simulink model "SD2231_Lab1_2022"  (R2020b)
settings: Solver=VariableStepAuto  StartTime=0.0  StopTime=inf  RelTol=1e-3
values from neighbouring files (symbols this model uses):
  delay = 250    [initial.m]
  K_awup = Ki_br_r/Kp_br_r    (= 10.4166666667)    [initial.m]
  K_brake = K_brake(3)    [initial.m]
  K_em = K_em(3)    [initial.m]
  Kd_br_f = 0*0.6*T_new_rl_b    (= 0)    [initial.m]
  Kd_br_r = 0.6*T_new_rl_b    (= 0.1722)    [initial.m]
  Kd_tr = 0.6*T_new    (= 0.0093)    [initial.m]
  Ki_br_f = 0.5*0.6*T_new_rl_b/L_new_rl_b^2    (= 37.3697916667)    [initial.m]
  Ki_br_r = 0.6*T_new_rl_b/L_new_rl_b^2    (= 74.7395833333)    [initial.m]
  Ki_tr = 0.6*T_new/L_new^2    (= 4.12188365651)    [initial.m]
  Kp_br_f = 1.2*T_new_rl_b/L_new_rl_b    (= 7.175)    [initial.m]
  Kp_br_r = 1.2*T_new_rl_b/L_new_rl_b    (= 7.175)    [initial.m]
  Kp_tr = 2.2*1.2*T_new/L_new    (= 0.861473684211)    [initial.m]
  N = 100    [initial.m]
  ref_br_f = 0.15    [initial.m]
  ref_br_r = 0.17-0.1    (= 0.07)    [initial.m]
  ref_tr = 0.06    [initial.m]
  step_time = 2    [initial.m]
  threshold_br_f = ref_br_f-0.05    (= 0.1)    [initial.m]
  threshold_br_r = ref_br_r-0.05    (= 0.02)    [initial.m]
  threshold_tc = ref_tr-0.02    (= 0.04)    [initial.m]
  vx_threshold = 1    [initial.m]
undefined symbols (not defined in the file or in its folder): DiscIntNeverNeededParam, Veh
libraries: CarMaker4SL x38, simulink x2, autolibmappedmotor x2
(part 2 of 4)

== system SD2231_Lab1_2022/CarMaker/Your ABS Controller/Activation Logic Br RR ==
  Brake Pedal : Inport
  vx : Inport  Port=2
  <Vehicle ax> : Inport  Port=3
  " Slip" : Inport  Port=4
  AdjBr FL : Scope  NumInputPorts=2
  Constant : Constant  Value=threshold_br_r
  Constant1 : Constant  Value=vx_threshold
  MATLAB Function : MATLAB Function  TreatAsAtomicUnit=on
  Subsystem : Subsystem
      settings: PortSchema="{\"entries\":[{\"content\":{\"sides\":[{\"content\":{\"connectorIds\":[\"In1\",\"In2\"]},\"type\":\"ConnectorPlacement.EquallySpacedRectSide\",\"uuid\":\"5cbd211e-f9c8-43f4-83d7-871b04fe90ea\"},{\"content\":{\"connectorIds\":[\"Out1\"],\"side\":\"RIGHT\"},\"type\":\"ConnectorPlacement.EquallySpacedRectSide\",\"uuid\":\"7fa8af9f-7b9f-4089-80e3-a9aa0072d831\"},{\"content\":{\"connectorIds\":[\"In3\"],\"side\":\"TOP\"},\"type\":\"ConnectorPlacement.EquallySpacedRectSide\",\"uuid\":\"e4a0fb24-cce3-4d5d-8c82-dcee69222b7b\"},{\"content\":{\"connectorIds\":[],\"side\":\"HIDDEN\"},\"type\":\"ConnectorPlacement.EquallySpacedRectSide\",\"uuid\":\"1dbaf2b9-056b-4908-bf5e-3fea819f12fb\"}]},\"type\":\"ConnectorPlacement.EquallySpacedConnector\",\"uuid\":\"c1423465-905b-4b91-a244-d319c117cff2\"}],\"packageUris\":[\"http://schema.mathworks.com/mf0/Connector/R2020b\"],\"version\":\"1.0\"}"
  ref : Constant  Value=ref_br_r
  BrkAdjust : Outport
  wires:
  Constant1/1 -> MATLAB Function/7(vx_threshold)
  ref/1 -> Subsystem/2(ref_slip)
  MATLAB Function/1(y) -> BrkAdjust/1, AdjBr FL/1
  Subsystem/1(AdjBr) -> MATLAB Function/5(AdjBrk)
  " Slip"/1 -> MATLAB Function/4(slip), Subsystem/1(slip)
  Brake Pedal/1 -> MATLAB Function/3(Brk), Subsystem/3(Brake Pedal), AdjBr FL/2
  Constant/1 -> MATLAB Function/6(threshold)
  <Vehicle ax>/1 -> MATLAB Function/2(ax)
  vx/1 -> MATLAB Function/1(vx)

== system SD2231_Lab1_2022/CarMaker/Your ABS Controller/Activation Logic Br RR old 2 ==
  Brake Pedal : Inport
  vx : Inport  Port=2
  <Vehicle ax> : Inport  Port=3
  " Slip" : Inport  Port=4
  AdjBr RR : Scope  NumInputPorts=2
  Constant : Constant  Value=threshold_br_r
  Constant1 : Constant  Value=vx_threshold
  Controller : Subsystem
      settings: PortSchema="{\"entries\":[{\"content\":{\"sides\":[{\"content\":{\"connectorIds\":[\"In1\",\"In2\"]},\"type\":\"ConnectorPlacement.EquallySpacedRectSide\",\"uuid\":\"5cec5cc2-4d6d-4b1d-b966-22042b341a0b\"},{\"content\":{\"connectorIds\":[\"Out1\"],\"side\":\"RIGHT\"},\"type\":\"ConnectorPlacement.EquallySpacedRectSide\",\"uuid\":\"00dd4905-e656-4dce-9ac4-4fe3f823c1f7\"},{\"content\":{\"connectorIds\":[\"In3\"],\"side\":\"TOP\"},\"type\":\"ConnectorPlacement.EquallySpacedRectSide\",\"uuid\":\"696fd126-3e4c-4262-b5bc-c3625537c515\"},{\"content\":{\"connectorIds\":[],\"side\":\"HIDDEN\"},\"type\":\"ConnectorPlacement.EquallySpacedRectSide\",\"uuid\":\"3dd45ed5-25e2-4347-abdf-21481b15662e\"}]},\"type\":\"ConnectorPlacement.EquallySpacedConnector\",\"uuid\":\"5000242c-67c6-4855-a207-79a064e97cc6\"}],\"packageUris\":[\"http://schema.mathworks.com/mf0/Connector/R2020b\"],\"version\":\"1.0\"}"
  MATLAB Function : MATLAB Function  TreatAsAtomicUnit=on
  Switch : Switch  Commented=on  Criteria=u2 > Threshold  Threshold=5
  ref : Constant  Value=ref_br_r
  ref1 : Constant  Commented=on  Value=0
  BrkAdjust : Outport
  tag scope: ref_br=global
  wires:
  <Vehicle ax>/1 -> MATLAB Function/2(ax)
  Constant/1 -> MATLAB Function/6(threshold)
  Brake Pedal/1 -> AdjBr RR/2, Controller/3(Brake Pedal), MATLAB Function/3(Brk)
  " Slip"/1 -> Controller/1(slip), MATLAB Function/4(slip)
  Controller/1(AdjThr) -> MATLAB Function/5(AdjBrk)
  MATLAB Function/1(y) -> BrkAdjust/1, AdjBr RR/1
  ref/1 -> Controller/2(ref_slip), [ref_br]
  vx/1 -> MATLAB Function/1(vx)
  Constant1/1 -> MATLAB Function/7(vx_threshold)
  ? -> Switch/2
  Switch/1 -> ?
  ref1/1 -> Switch/3

== system SD2231_Lab1_2022/CarMaker/Your ABS Controller/Activation Logic1 ==
  Brake Pedal : Inport
  vx : Inport  Port=2
  <Vehicle ax> : Inport  Port=3
  " Slip" : Inport  Port=4
  Constant : Constant  Value=threshold_br_f
  MATLAB Function : MATLAB Function  Commented=on  TreatAsAtomicUnit=on
  MATLAB Function1 : MATLAB Function  TreatAsAtomicUnit=on
  Scope : Scope
  Scope1 : Scope
  Subsystem : Subsystem  Commented=on
  Subsystem1 : Subsystem
      settings: PortSchema="{\"entries\":[{\"content\":{\"sides\":[{\"content\":{\"connectorIds\":[\"In1\",\"In2\"]},\"type\":\"ConnectorPlacement.EquallySpacedRectSide\",\"uuid\":\"8c5c4b92-db61-456f-8d74-c8cf023ef126\"},{\"content\":{\"connectorIds\":[\"Out1\"],\"side\":\"RIGHT\"},\"type\":\"ConnectorPlacement.EquallySpacedRectSide\",\"uuid\":\"6d2f9992-79bb-457d-890b-805505bdee0e\"},{\"content\":{\"connectorIds\":[],\"side\":\"TOP\"},\"type\":\"ConnectorPlacement.EquallySpacedRectSide\",\"uuid\":\"0d630a28-683f-44cf-bfe5-2a203886c9bc\"},{\"content\":{\"connectorIds\":[\"In3\"],\"side\":\"BOTTOM\"},\"type\":\"ConnectorPlacement.EquallySpacedRectSide\",\"uuid\":\"65c4d467-3a6d-4ab0-8a2a-27ecddcdb5a7\"},{\"content\":{\"connectorIds\":[],\"side\":\"HIDDEN\"},\"type\":\"ConnectorPlacement.EquallySpacedRectSide\",\"uuid\":\"17dfa9f0-a896-4b0a-816c-6439308f7c21\"}]},\"type\":\"ConnectorPlacement.EquallySpacedConnector\",\"uuid\":\"38ebf0b2-c1be-4567-9f2f-ae9c854cb505\"}],\"packageUris\":[\"http://schema.mathworks.com/mf0/Connector/R2020b\"],\"version\":\"1.0\"}"
  Switch : Switch  Criteria=u2 > Threshold  Threshold=0.5
  ref : Constant  Value=ref_br_f
  BrkAdjust : Outport
  wires:
  Constant/1 -> MATLAB Function1/4(threshold)
  ref/1 -> Subsystem1/2(ref_slip)
  MATLAB Function1/1(s) -> Subsystem1/1(slip)
  " Slip"/1 -> MATLAB Function1/3(slip)
  MATLAB Function1/2(y) -> Scope/1, Subsystem1/3(y), Switch/2
  Brake Pedal/1 -> Switch/3, MATLAB Function1/5(Brk)
  Subsystem/1(AdjThr) -> MATLAB Function/5(AdjBrk)
  <Vehicle ax>/1 -> MATLAB Function1/1(ax)
  vx/1 -> MATLAB Function1/2(vx)
  ? -> Subsystem/1(slip), MATLAB Function/4(slip)
  Subsystem1/1(AdjThr) -> Switch/1
  Switch/1 -> Scope1/1, BrkAdjust/1

== system SD2231_Lab1_2022/CarMaker/Your Traction Controller/Activation Logic RL tr1 ==
  Thr : Inport
  vx : Inport  Port=2
  <Vehicle ax> : Inport  Port=3
  " Slip" : Inport  Port=4
  Constant : Constant  Value=threshold_tc
  If : If  IfExpression=u1 > 0.5
  If Action Subsystem : Subsystem  TreatAsAtomicUnit=on
  MATLAB Function : MATLAB Function  Commented=on  TreatAsAtomicUnit=on
  MATLAB Function1 : MATLAB Function  TreatAsAtomicUnit=on
  Merge : Merge
  Scope : Scope
  Scope1 : Scope
  Subsystem : Subsystem  Commented=on
  Subsystem1 : Subsystem
  ref : Constant  Value=ref_tr
  y tracking RL tr : Scope
  AdjThr : Outport
  wires:
  Merge/1 -> AdjThr/1, Scope/1
  If Action Subsystem/1(Out1) -> Merge/2
  If/2 -> If Action Subsystem/Action
  If/1 -> Subsystem1/Action
  Subsystem1/1(AdjThr) -> Merge/1
  ? -> MATLAB Function/4(slip), Subsystem/1(slip)
  vx/1 -> MATLAB Function1/2(vx)
  <Vehicle ax>/1 -> MATLAB Function1/1(ax)
  Subsystem/1(AdjThr) -> MATLAB Function/5(AdjBrk)
  Thr/1 -> MATLAB Function1/5(Thr), Subsystem1/3(Thr), If Action Subsystem/1(Throttle), Scope1/1
  MATLAB Function1/2(y) -> If/1, y tracking RL tr/1
  " Slip"/1 -> MATLAB Function1/3(slip)
  MATLAB Function1/1(s) -> Subsystem1/1(slip)
  ref/1 -> Subsystem1/2(ref_slip)
  Constant/1 -> MATLAB Function1/4(threshold)

== system SD2231_Lab1_2022/CarMaker/Your Traction Controller/Activation Logic RL tr2 ==
  Thr : Inport
  vx : Inport  Port=2
  <Vehicle ax> : Inport  Port=3
  " Slip" : Inport  Port=4
  Add : Sum
  Constant : Constant  Value=threshold_tc
  MATLAB Function : MATLAB Function  Commented=on  TreatAsAtomicUnit=on
  MATLAB Function1 : MATLAB Function  TreatAsAtomicUnit=on
  Subsystem : Subsystem  Commented=on
  Subsystem2 : Subsystem
  ref1 : Constant  Value=ref_tr
  AdjThr : Outport
  wires:
  ? -> MATLAB Function/4(slip), Subsystem/1(slip)
  vx/1 -> MATLAB Function1/2(vx)
  <Vehicle ax>/1 -> MATLAB Function1/1(ax)
  Subsystem/1(AdjThr) -> MATLAB Function/5(AdjBrk)
  Thr/1 -> Add/2, MATLAB Function1/5(Thr)
  " Slip"/1 -> MATLAB Function1/3(slip)
  Constant/1 -> MATLAB Function1/4(threshold)
  ref1/1 -> Subsystem2/2(ref_slip)
  Subsystem2/1(AdjThr) -> Add/1
  Add/1 -> AdjThr/1
  ? -> Subsystem2/1(slip)

== system SD2231_Lab1_2022/CarMaker/Your Traction Controller/Activation Logic Tr RL ==
  <Throttle> : Inport
  ax : Inport  Port=2
  <RL Slip> : Inport  Port=3
  AdjTh RL : Scope
  Constant : Constant  Value=threshold_tc
  Delay : Delay  Commented=on  DelayLength=delay
  MATLAB Function : MATLAB Function  TreatAsAtomicUnit=on
  Subsystem : Subsystem
      settings: PortSchema="{\"entries\":[{\"content\":{\"sides\":[{\"content\":{\"connectorIds\":[\"In1\",\"In2\"]},\"type\":\"ConnectorPlacement.EquallySpacedRectSide\",\"uuid\":\"79f5dd27-5b3e-419d-80a6-0989bf4121ab\"},{\"content\":{\"connectorIds\":[\"Out1\"],\"side\":\"RIGHT\"},\"type\":\"ConnectorPlacement.EquallySpacedRectSide\",\"uuid\":\"49c92f03-337c-4fd9-9025-501eb5f091b3\"},{\"content\":{\"connectorIds\":[\"In3\"],\"side\":\"TOP\"},\"type\":\"ConnectorPlacement.EquallySpacedRectSide\",\"uuid\":\"f0086f1c-5e21-497a-b605-cecce1a91be6\"},{\"content\":{\"connectorIds\":[],\"side\":\"HIDDEN\"},\"type\":\"ConnectorPlacement.EquallySpacedRectSide\",\"uuid\":\"c7823733-75a9-46f7-a877-dbd7359ce4af\"}]},\"type\":\"ConnectorPlacement.EquallySpacedConnector\",\"uuid\":\"cd50cf1a-1747-4545-b326-76b9fad2c095\"}],\"packageUris\":[\"http://schema.mathworks.com/mf0/Connector/R2020b\"],\"version\":\"1.0\"}"
  ref : Constant  Value=ref_tr
  y tracking RR : Scope
  RLTrqAdjust : Outport
  wires:
  Subsystem/1(AdjThr) -> MATLAB Function/4(AdjThr)
  MATLAB Function/2(dbg) -> y tracking RR/1
  ax/1 -> MATLAB Function/1(ax)
  Constant/1 -> MATLAB Function/5(threshold)
  <Throttle>/1 -> Subsystem/3(<Throttle>), MATLAB Function/2(Thr)
  <RL Slip>/1 -> Subsystem/1(slip), MATLAB Function/3(slip)
  MATLAB Function/1(y) -> AdjTh RL/1, RLTrqAdjust/1
  ref/1 -> Subsystem/2(ref_slip)

== system SD2231_Lab1_2022/CarMaker/Your Traction Controller/Activation Logic Tr RR ==
  Thr : Inport
  <Vehicle ax> : Inport  Port=2
  " Slip" : Inport  Port=3
  AdjTh RR : Scope
  Constant : Constant  Value=threshold_tc
  Controller : Subsystem  Commented=on
      settings: PortSchema="{\"entries\":[{\"content\":{\"sides\":[{\"content\":{\"connectorIds\":[\"In1\",\"In2\"]},\"type\":\"ConnectorPlacement.EquallySpacedRectSide\",\"uuid\":\"52813697-ab49-4c87-b189-f3c4bbd3a435\"},{\"content\":{\"connectorIds\":[\"Out1\"],\"side\":\"RIGHT\"},\"type\":\"ConnectorPlacement.EquallySpacedRectSide\",\"uuid\":\"31f7970c-8430-4628-a4a3-49e1cbd89ba0\"},{\"content\":{\"connectorIds\":[\"In3\"],\"side\":\"TOP\"},\"type\":\"ConnectorPlacement.EquallySpacedRectSide\",\"uuid\":\"62e35f04-27eb-4615-837d-613f48d08a05\"},{\"content\":{\"connectorIds\":[],\"side\":\"HIDDEN\"},\"type\":\"ConnectorPlacement.EquallySpacedRectSide\",\"uuid\":\"731c0a9f-c9f4-41b7-8d96-4f2cebcab437\"}]},\"type\":\"ConnectorPlacement.EquallySpacedConnector\",\"uuid\":\"9bef8a7f-94a8-4a01-95b1-5b9f04346e26\"}],\"packageUris\":[\"http://schema.mathworks.com/mf0/Connector/R2020b\"],\"version\":\"1.0\"}"
  MATLAB Function : MATLAB Function  TreatAsAtomicUnit=on
  Subsystem : Subsystem
      settings: PortSchema="{\"entries\":[{\"content\":{\"sides\":[{\"content\":{\"connectorIds\":[\"In1\",\"In2\"]},\"type\":\"ConnectorPlacement.EquallySpacedRectSide\",\"uuid\":\"79f5dd27-5b3e-419d-80a6-0989bf4121ab\"},{\"content\":{\"connectorIds\":[\"Out1\"],\"side\":\"RIGHT\"},\"type\":\"ConnectorPlacement.EquallySpacedRectSide\",\"uuid\":\"49c92f03-337c-4fd9-9025-501eb5f091b3\"},{\"content\":{\"connectorIds\":[\"In3\"],\"side\":\"TOP\"},\"type\":\"ConnectorPlacement.EquallySpacedRectSide\",\"uuid\":\"f0086f1c-5e21-497a-b605-cecce1a91be6\"},{\"content\":{\"connectorIds\":[],\"side\":\"HIDDEN\"},\"type\":\"ConnectorPlacement.EquallySpacedRectSide\",\"uuid\":\"c7823733-75a9-46f7-a877-dbd7359ce4af\"}]},\"type\":\"ConnectorPlacement.EquallySpacedConnector\",\"uuid\":\"cd50cf1a-1747-4545-b326-76b9fad2c095\"}],\"packageUris\":[\"http://schema.mathworks.com/mf0/Connector/R2020b\"],\"version\":\"1.0\"}"
  ref : Constant  Value=ref_tr
  ThrAdjust : Outport
  wires:
  <Vehicle ax>/1 -> MATLAB Function/1(ax)
  Constant/1 -> MATLAB Function/5(threshold)
  Thr/1 -> Subsystem/3(<Throttle>), MATLAB Function/2(Thr)
  " Slip"/1 -> Subsystem/1(slip), MATLAB Function/3(slip)
  Subsystem/1(AdjThr) -> MATLAB Function/4(AdjThr)
  MATLAB Function/1(y) -> AdjTh RR/1, ThrAdjust/1
  ref/1 -> Subsystem/2(ref_slip)

== system SD2231_Lab1_2022/CarMaker/Your Traction Controller/Activation Logic1 ==
  <Throttle> : Inport
  <Vehicle ax> : Inport  Port=2
  <RL Slip> : Inport  Port=3
  Constant : Constant  Value=threshold_tc
  MATLAB Function : MATLAB Function  TreatAsAtomicUnit=on
  Subsystem : Subsystem
  ref : Constant  Value=ref_tr
  TrqAdjust : Outport
  wires:
  <Throttle>/1 -> MATLAB Function/2(Thr)
  <RL Slip>/1 -> Subsystem/1(slip), MATLAB Function/3(slip)
  Subsystem/1(AdjThr) -> MATLAB Function/4(AdjThr)
  ref/1 -> Subsystem/2(ref_slip)
  Constant/1 -> MATLAB Function/5(threshold)
  MATLAB Function/1(y) -> TrqAdjust/1
  <Vehicle ax>/1 -> MATLAB Function/1(ax)

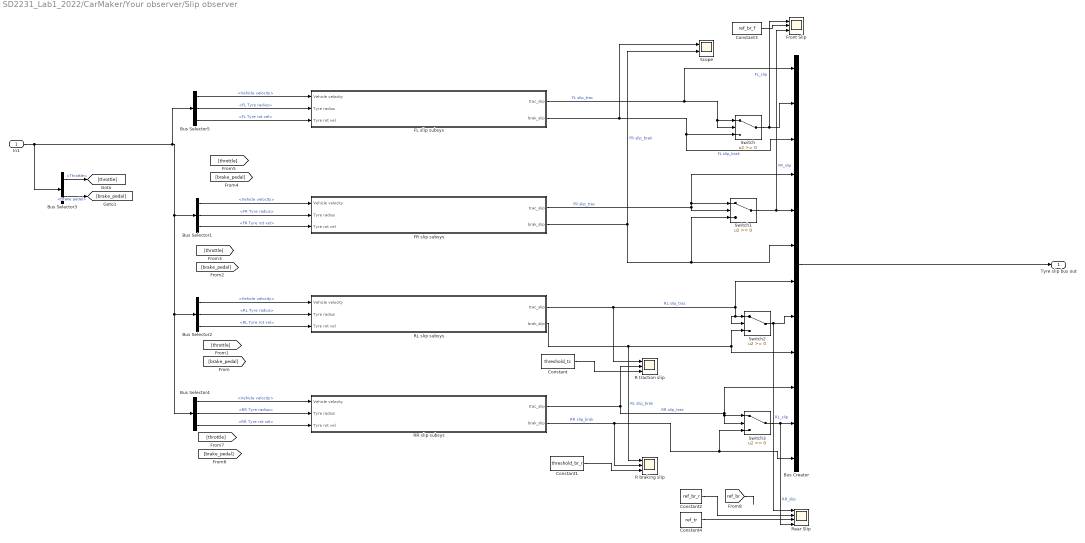
== system SD2231_Lab1_2022/CarMaker/Your observer/Slip observer ==
  In1 : Inport
  " FL slip subsys" : Subsystem
  " FR slip subsys" : Subsystem
  " RL slip subsys" : Subsystem
  " RR slip subsys" : Subsystem
  Bus Creator : BusCreator  Inputs=12
  Bus Selector1 : BusSelector  OutputSignals=Vehicle velocity,FR Tyre radius,FR Tyre rot vel
  Bus Selector2 : BusSelector  OutputSignals=Vehicle velocity,RL Tyre radius,RL Tyre rot vel
  Bus Selector3 : BusSelector  OutputSignals=Throttle,Brake pedal
  Bus Selector4 : BusSelector  OutputSignals=Vehicle velocity,RR Tyre radius,RR Tyre rot vel
  Bus Selector5 : BusSelector  OutputSignals=Vehicle velocity,FL Tyre radius,FL Tyre rot vel
  Constant : Constant  Value=threshold_tc
  Constant1 : Constant  Value=threshold_br_r
  Constant2 : Constant  Value=ref_br_r
  Constant3 : Constant  Value=ref_br_f
  Constant4 : Constant  Value=ref_tr
  Front Slip : Scope  NumInputPorts=3
  R braking slip : Scope  NumInputPorts=3
  R traction slip : Scope  NumInputPorts=3
  Rear Slip : Scope  NumInputPorts=4
  Scope : Scope  NumInputPorts=2
  Switch{,1..3} (4 alike) : Switch
  Tyre slip bus out : Outport
  wires:
  Bus Selector3/1 -> [throttle]  "<Throttle>"
  Bus Selector3/2 -> [brake_pedal]  "<Brake pedal>"
  Bus Selector4/1 -> " RR slip subsys"/1(Vehicle velocity)  "<Vehicle velocity>"
  Bus Selector4/2 -> " RR slip subsys"/2(" Tyre radius")  "<RR Tyre radius>"
  Bus Selector4/3 -> " RR slip subsys"/3(Tyre rot vel)  "<RR Tyre rot vel>"
  " FL slip subsys"/1(trac_slip) -> Switch/2, Switch/1, Bus Creator/1  "FL slip_trac"
  " FL slip subsys"/2(brak_slip) -> Scope/1, Bus Creator/3, Switch/3  "FL slip_brak"
  " RL slip subsys"/2(brak_slip) -> R braking slip/1, Bus Creator/9, Switch2/3  "RL slip_brak"
  " RL slip subsys"/1(trac_slip) -> Switch2/2, Switch2/1, Bus Creator/7, R traction slip/1  "RL slip_trac"
  " RR slip subsys"/1(trac_slip) -> R traction slip/2, Switch3/2, Switch3/1, Bus Creator/10  "RR slip_trac"
  " RR slip subsys"/2(brak_slip) -> R braking slip/2, Switch3/3, Bus Creator/12  "RR slip_brak"
  Bus Selector2/1 -> " RL slip subsys"/1(Vehicle velocity)  "<Vehicle velocity>"
  Bus Selector2/2 -> " RL slip subsys"/2(" Tyre radius")  "<RL Tyre radius>"
  Bus Selector2/3 -> " RL slip subsys"/3(Tyre rot vel)  "<RL Tyre rot vel>"
  Bus Selector1/2 -> " FR slip subsys"/2(" Tyre radius")  "<FR Tyre radius>"
  Bus Selector1/1 -> " FR slip subsys"/1(Vehicle velocity)  "<Vehicle velocity>"
  Bus Selector1/3 -> " FR slip subsys"/3(Tyre rot vel)  "<FR Tyre rot vel>"
  " FR slip subsys"/2(brak_slip) -> Scope/2, Switch1/3, Bus Creator/6  "FR slip_brak"
  " FR slip subsys"/1(trac_slip) -> Bus Creator/4, Switch1/1, Switch1/2  "FR slip_trac"
  Bus Selector5/3 -> " FL slip subsys"/3(Tyre rot vel)  "<FL Tyre rot vel>"
  In1/1 -> Bus Selector3/1, Bus Selector5/1, Bus Selector1/1, Bus Selector4/1, Bus Selector2/1
  Bus Selector5/1 -> " FL slip subsys"/1(Vehicle velocity)  "<Vehicle velocity>"
  Bus Selector5/2 -> " FL slip subsys"/2(" Tyre radius")  "<FL Tyre radius>"
  Constant/1 -> R traction slip/3
  Switch/1 -> Front Slip/1, Bus Creator/2  "FL_slip"
  Switch1/1 -> Front Slip/3, Bus Creator/5  "FR_slip"
  Switch2/1 -> Rear Slip/1, Bus Creator/8  "RL_slip"
  Switch3/1 -> Rear Slip/4, Bus Creator/11  "RR_slip"
  Bus Creator/1 -> Tyre slip bus out/1
  Constant1/1 -> R braking slip/3
  Constant4/1 -> Rear Slip/3
  [ref_br] -> ?
  Constant3/1 -> Front Slip/2
  Constant2/1 -> Rear Slip/2

== system SD2231_Lab1_2022/CarMaker/IPG Vehicle/Brake/CreateBus Vhcl.Wheel.PT ==
  In : Inport
  BusCreator1 : BusCreator  Inputs=20
  Demux1 : Demux  Outputs=20
      settings: DisplayOption=none
  Out : Outport
  wires:
  Demux1/20 -> BusCreator1/20  "Vhcl Trq_DriveSrc_trg d3"
  Demux1/19 -> BusCreator1/19  "Vhcl Trq_DriveSrc_trg d2"
  Demux1/18 -> BusCreator1/18  "Vhcl Trq_DriveSrc_trg d1"
  Demux1/17 -> BusCreator1/17  "Vhcl Trq_DriveSrc_trg d0"
  Demux1/16 -> BusCreator1/16  "Vhcl Wheel RR WhlBearing"
  Demux1/15 -> BusCreator1/15  "Vhcl Wheel RR Trq_T2W"
  Demux1/14 -> BusCreator1/14  "Vhcl Wheel RR Trq_BrakeReg_trg"
  Demux1/13 -> BusCreator1/13  "Vhcl Wheel RR Trq_Brake"
  Demux1/12 -> BusCreator1/12  "Vhcl Wheel RL WhlBearing"
  Demux1/11 -> BusCreator1/11  "Vhcl Wheel RL Trq_T2W"
  Demux1/10 -> BusCreator1/10  "Vhcl Wheel RL Trq_BrakeReg_trg"
  Demux1/9 -> BusCreator1/9  "Vhcl Wheel RL Trq_Brake"
  Demux1/8 -> BusCreator1/8  "Vhcl Wheel FR WhlBearing"
  Demux1/7 -> BusCreator1/7  "Vhcl Wheel FR Trq_T2W"
  Demux1/6 -> BusCreator1/6  "Vhcl Wheel FR Trq_BrakeReg_trg"
  Demux1/5 -> BusCreator1/5  "Vhcl Wheel FR Trq_Brake"
  Demux1/4 -> BusCreator1/4  "Vhcl Wheel FL WhlBearing"
  Demux1/3 -> BusCreator1/3  "Vhcl Wheel FL Trq_T2W"
  Demux1/2 -> BusCreator1/2  "Vhcl Wheel FL Trq_BrakeReg_trg"
  Demux1/1 -> BusCreator1/1  "Vhcl Wheel FL Trq_Brake"
  BusCreator1/1 -> Out/1
  In/1 -> Demux1/1

== system SD2231_Lab1_2022/CarMaker/IPG Vehicle/Brake/UserDefinedBrakingSystem ==
  note: Please note: Influence of DrivMan.Handbrake on the braking
      | torques (Brake IF Trq_XX signals) is ignored in this example.
  SD2231.Data : Inport
  Bus Creator2 : BusCreator  Inputs=16
  Bus Selector : BusSelector  OutputSignals=FLBrakeAdjust,FRBrakeAdjust,RLBrakeAdjust,RRBrakeAdjust
  Constant : Constant  Value=0
  NOTSET : Constant  Value=-99999
  Subsystem : Subsystem
  Subsystem1 : Subsystem
  Subsystem2 : Subsystem
  Subsystem3 : Subsystem
  Brake.IF.Out : Outport  VectorParamsAs1DForOutWhenUnconnected=off
  wires:
  SD2231.Data/1 -> Bus Selector/1
  Bus Creator2/1 -> Brake.IF.Out/1
  Constant/1 -> Bus Creator2/10, Bus Creator2/5, Bus Creator2/6, Bus Creator2/7, Bus Creator2/8, Bus Creator2/9, Bus Creator2/11, Bus Creator2/12
  NOTSET/1 -> Bus Creator2/13, Bus Creator2/14, Bus Creator2/15, Bus Creator2/16
  Subsystem/1(FL brake force) -> Bus Creator2/1
  Bus Selector/1 -> Subsystem/1(FLBrakeAdjust)  "<FLBrakeAdjust>"
  Subsystem1/1(FR brake force) -> Bus Creator2/2
  Subsystem2/1(RL brake force) -> Bus Creator2/3
  Subsystem3/1(RR brake force) -> Bus Creator2/4
  Bus Selector/2 -> Subsystem1/1(FRBrakeAdjust)  "<FRBrakeAdjust>"
  Bus Selector/3 -> Subsystem2/1(RLBrakeAdjust)  "<RLBrakeAdjust>"
  Bus Selector/4 -> Subsystem3/1(RRBrakeAdjust)  "<RRBrakeAdjust>"

== system SD2231_Lab1_2022/CarMaker/IPG Vehicle/CarAndTrailer/CarAndTrailerUpd ==
  Sync_In : Inport
  Vhcl.Steering : Inport  Port=2
  Vhcl.Motion : Inport  Port=3
  Vhcl.PoI : Inport  Port=4
  Vhcl.Wheel.FL : Inport  Port=5
  Vhcl.Wheel.FR : Inport  Port=6
  Vhcl.Wheel.RL : Inport  Port=7
  Vhcl.Wheel.RR : Inport  Port=8
  Car.Hitch.FrcTrq : Inport  Port=9
  Vhcl.Fr1A : Inport  Port=10
  CarAndTrailerUpd : S-Function  FunctionName=CM_Sfun  Parameters='CarAndTrUpd'  SFunctionDeploymentMode=off  EnableBusSupport=off
  CreateBus Brake.IF.In : Subsystem
  Sync_Out : Outport
  Brake.IF.In : Outport  Port=2
  wires:
  Vhcl.Fr1A/1 -> CarAndTrailerUpd/10  "user vehicle only"
  Vhcl.Steering/1 -> CarAndTrailerUpd/2
  Vhcl.Motion/1 -> CarAndTrailerUpd/3
  Vhcl.PoI/1 -> CarAndTrailerUpd/4
  Vhcl.Wheel.FL/1 -> CarAndTrailerUpd/5
  Vhcl.Wheel.FR/1 -> CarAndTrailerUpd/6
  Car.Hitch.FrcTrq/1 -> CarAndTrailerUpd/9
  Vhcl.Wheel.RR/1 -> CarAndTrailerUpd/8
  Vhcl.Wheel.RL/1 -> CarAndTrailerUpd/7
  CarAndTrailerUpd/2 -> CreateBus Brake.IF.In/1(In)
  CreateBus Brake.IF.In/1(Out) -> Brake.IF.In/1
  CarAndTrailerUpd/1 -> Sync_Out/1
  Sync_In/1 -> CarAndTrailerUpd/1

== system SD2231_Lab1_2022/CarMaker/IPG Vehicle/CarAndTrailer/Forces ==
  Sync_In : Inport
  TireFL_In : Inport  Port=2
  TireFR_In : Inport  Port=3
  TireRL_In : Inport  Port=4
  TireRR_In : Inport  Port=5
  lSpring : Inport  Port=6
  vDamp : Inport  Port=7
  lStabi : Inport  Port=8
  lBuf : Inport  Port=9
  External Suspension Forces : Subsystem
  Suspension Forces : Subsystem
  Tires : Subsystem
  Vehicle Forces : Subsystem
  Sync_Out : Outport
  Car.Virtual : Outport  Port=2
  Car.Aero : Outport  Port=3
  Car.Load : Outport  Port=4
  TireFL_Out : Outport  Port=5
  TireFR_Out : Outport  Port=6
  TireRL_Out : Outport  Port=7
  TireRR_Out : Outport  Port=8
  FSpring_ext : Outport  Port=9
  FDamp_ext : Outport  Port=10
  FStabi_ext : Outport  Port=11
  FBuf_ext : Outport  Port=12
  wires:
  lBuf/1 -> External Suspension Forces/5(lBuf), Suspension Forces/5(lBuf)
  lStabi/1 -> External Suspension Forces/4(lStabi), Suspension Forces/4(lStabi)
  vDamp/1 -> External Suspension Forces/3(vDamp), Suspension Forces/3(vDamp)
  Tires/4(TireRR_Out) -> TireRR_Out/1
  Tires/3(TireRL_Out) -> TireRL_Out/1
  Tires/2(TireFR_Out) -> TireFR_Out/1
  Tires/1(TireFL_Out) -> TireFL_Out/1
  TireRR_In/1 -> Tires/5(TireRR_In)
  TireRL_In/1 -> Tires/4(TireRL_In)
  TireFR_In/1 -> Tires/3(TireFR_In)
  TireFL_In/1 -> Tires/2(TireFL_In)
  External Suspension Forces/4(FBuf_ext) -> FBuf_ext/1
  Sync_In/1 -> External Suspension Forces/1(Sync_In), Tires/1(Sync_In), Vehicle Forces/1(Sync_In)
  Vehicle Forces/1(Sync_Out) -> Suspension Forces/1(Sync_In)
  Vehicle Forces/2(Car.Virtual) -> Car.Virtual/1
  Vehicle Forces/3(Car.Aero) -> Car.Aero/1
  Vehicle Forces/4(Car.Load) -> Car.Load/1
  lSpring/1 -> External Suspension Forces/2(lSpring), Suspension Forces/2(lSpring)
  External Suspension Forces/2(FDamp_ext) -> FDamp_ext/1
  External Suspension Forces/3(FStabi_ext) -> FStabi_ext/1
  External Suspension Forces/1(FSpring_ext) -> FSpring_ext/1
  Suspension Forces/1(Sync_Out) -> Sync_Out/1

== system SD2231_Lab1_2022/CarMaker/IPG Vehicle/CarAndTrailer/Kinematics ==
  Sync_In : Inport
  Steer.IF : Inport  Port=2
  Kinematics : S-Function  FunctionName=CM_Sfun  Parameters='Kinematics'  SFunctionDeploymentMode=off  EnableBusSupport=off
  Sync_Out : Outport
  TireFL_In : Outport  Port=2
  TireFR_In : Outport  Port=3
  TireRL_In : Outport  Port=4
  TireRR_In : Outport  Port=5
  lSpring : Outport  Port=6
  vDamp : Outport  Port=7
  lStabi : Outport  Port=8
  lBuf : Outport  Port=9
  wires:
  Kinematics/9 -> lBuf/1
  Kinematics/8 -> lStabi/1
  Kinematics/2 -> TireFL_In/1
  Kinematics/3 -> TireFR_In/1
  Kinematics/4 -> TireRL_In/1
  Kinematics/5 -> TireRR_In/1
  Kinematics/6 -> lSpring/1
  Kinematics/7 -> vDamp/1
  Sync_In/1 -> Kinematics/1
  Kinematics/1 -> Sync_Out/1
  Steer.IF/1 -> Kinematics/2

== system SD2231_Lab1_2022/CarMaker/IPG Vehicle/CarAndTrailer/Kinetics ==
  Sync_In : Inport
  Car.Virtual : Inport  Port=2
  Car.Aero : Inport  Port=3
  Car.Load : Inport  Port=4
  TireFL.Out : Inport  Port=5
  TireFR.Out : Inport  Port=6
  TireRL.Out : Inport  Port=7
  TireRR.Out : Inport  Port=8
  FSpring_ext : Inport  Port=9
  FDamp_ext : Inport  Port=10
  FStabi_ext : Inport  Port=11
  FBuf_ext : Inport  Port=12
  Bus Creator : BusCreator  Inputs=4
  Bus Creator1 : BusCreator  Inputs=12
  Bus Creator2 : BusCreator  Inputs=6
  Bus Creator3 : BusCreator  Inputs=6
  Bus Creator4 : BusCreator  Inputs=4
  Demux : Demux  Outputs=12
      settings: DisplayOption=none
  Demux1 : Demux  Outputs=6
      settings: DisplayOption=none
  Demux2 : Demux  Outputs=6
      settings: DisplayOption=none
  Demux3 : Demux
      settings: DisplayOption=none
  Demux4 : Demux
      settings: DisplayOption=none
  Kinetics : S-Function  FunctionName=CM_Sfun  Parameters='Kinetics'  SFunctionDeploymentMode=off  EnableBusSupport=off
  Sync_Out : Outport
  Trailer.Load : Outport  Port=2
  Car.Hitch : Outport  Port=3
  Car.Fr1 : Outport  Port=4
  Car.Trq_T2W : Outport  Port=5
  WheelCarrier.Misc : Outport  Port=6
  wires:
  FBuf_ext/1 -> Kinetics/12
  Sync_In/1 -> Kinetics/1
  Kinetics/1 -> Sync_Out/1
  Car.Aero/1 -> Kinetics/3
  Car.Virtual/1 -> Kinetics/2
  Bus Creator1/1 -> Trailer.Load/1
  Demux/1 -> Bus Creator1/1  "Trailer Load_0 mass"
  Demux/2 -> Bus Creator1/2  "Trailer Load_0 tx"
  Demux/3 -> Bus Creator1/3  "Trailer Load_0 ty"
  Demux/4 -> Bus Creator1/4  "Trailer Load_0 tz"
  Kinetics/2 -> Demux/1
  Demux/5 -> Bus Creator1/5  "Trailer Load_1 mass"
  Demux/6 -> Bus Creator1/6  "Trailer Load_1 tx"
  Demux/7 -> Bus Creator1/7  "Trailer Load_1 ty"
  Demux/8 -> Bus Creator1/8  "Trailer Load_1 tz"
  Demux/9 -> Bus Creator1/9  "Trailer Load_2 mass"
  Demux/10 -> Bus Creator1/10  "Trailer Load_2 tx"
  Demux/11 -> Bus Creator1/11  "Trailer Load_2 ty"
  Demux/12 -> Bus Creator1/12  "Trailer Load_2 tz"
  Demux1/1 -> Bus Creator2/1  "Car Hitch tx"
  Demux1/2 -> Bus Creator2/2  "Car Hitch ty"
  Demux1/3 -> Bus Creator2/3  "Car Hitch tz"
  Demux1/4 -> Bus Creator2/4  "Car Hitch vx"
  Demux1/5 -> Bus Creator2/5  "Car Hitch vy"
  Demux1/6 -> Bus Creator2/6  "Car Hitch vz"
  Kinetics/3 -> Demux1/1
  Bus Creator2/1 -> Car.Hitch/1
  Demux2/1 -> Bus Creator3/1  "Car Fr1 rx"
  Demux2/2 -> Bus Creator3/2  "Car Fr1 ry"
  Demux2/3 -> Bus Creator3/3  "Car Fr1 rz"
  Demux2/4 -> Bus Creator3/4  "Car Fr1 rvx"
  Demux2/5 -> Bus Creator3/5  "Car Fr1 rvy"
  Demux2/6 -> Bus Creator3/6  "Car Fr1 rvz"
  Bus Creator3/1 -> Car.Fr1/1
  Kinetics/4 -> Demux2/1
  Car.Load/1 -> Kinetics/4
  Demux3/1 -> Bus Creator4/1  "car Susp FL GenInert2"
  Demux3/2 -> Bus Creator4/2  "car Susp FR GenInert2"
  Demux3/3 -> Bus Creator4/3  "car Susp FL GenFrc2"
  Demux3/4 -> Bus Creator4/4  "car Susp FR GenFrc2"
  Bus Creator4/1 -> WheelCarrier.Misc/1
  Bus Creator/1 -> Car.Trq_T2W/1
  Demux4/4 -> Bus Creator/4  "Car Trq_T2WRR"
  Demux4/3 -> Bus Creator/3  "Car Trq_T2WRL"
  Demux4/2 -> Bus Creator/2  "Car Trq_T2WFR"
  Demux4/1 -> Bus Creator/1  "Car Trq_T2WFL"
  TireFL.Out/1 -> Kinetics/5
  TireFR.Out/1 -> Kinetics/6
  TireRL.Out/1 -> Kinetics/7
  TireRR.Out/1 -> Kinetics/8
  FSpring_ext/1 -> Kinetics/9
  FDamp_ext/1 -> Kinetics/10
  FStabi_ext/1 -> Kinetics/11
  Kinetics/6 -> Demux3/1
  Kinetics/5 -> Demux4/1

== system SD2231_Lab1_2022/CarMaker/IPG Vehicle/CarAndTrailer/Steering ==
  note: When replacing the entire steering system,
      | be sure to disable the IPG steering model by using the steering
      | model 'Model Manager off' in the vehicle GUI.
  Sync_In : Inport
  VhclCtrl.Steering : Inport  Port=2
  Bus Creator1 : BusCreator  Inputs=16
  Bus Creator2 : BusCreator  Inputs=5
  Demux : Demux  Outputs=21
      settings: DisplayOption=none
  Steering : S-Function  FunctionName=CM_Sfun  Parameters='Steering'  SFunctionDeploymentMode=off  EnableBusSupport=off
  Terminator : Terminator
  Sync_Out : Outport
  Steer.IF : Outport  Port=2
  wires:
  Demux/21 -> Bus Creator2/5  "Steering IF R Inert"
  Demux/20 -> Bus Creator2/4  "Steering IF R Frc"
  Demux/19 -> Bus Creator2/3  "Steering IF L Inert"
  Demux/18 -> Bus Creator2/2  "Steering IF L Frc"
  Demux/17 -> Bus Creator2/1  "Steering IF SteerByTrq"
  Demux/16 -> Bus Creator1/16  "Steering IF R iSteer2q"
  Demux/15 -> Bus Creator1/15  "Steering IF R qpp"
  Demux/14 -> Bus Creator1/14  "Steering IF R qp"
  Demux/13 -> Bus Creator1/13  "Steering IF R q"
  Demux/12 -> Bus Creator1/12  "Steering IF L iSteer2q"
  Demux/11 -> Bus Creator1/11  "Steering IF L qpp"
  Demux/10 -> Bus Creator1/10  "Steering IF L qp"
  Demux/9 -> Bus Creator1/9  "Steering IF L q"
  Demux/8 -> Bus Creator1/8  "Steering IF AssistTrqPin"
  Demux/7 -> Bus Creator1/7  "Steering IF AssistTrqCol"
  Demux/6 -> Bus Creator1/6  "Steering IF AssistFrc"
  Demux/5 -> Bus Creator1/5  "Steering IF TrqStatic"
  Demux/4 -> Bus Creator1/4  "Steering IF Trq"
  Demux/3 -> Bus Creator1/3  "Steering IF AngAcc"
  Demux/2 -> Bus Creator1/2  "Steering IF AngVel"
  Demux/1 -> Bus Creator1/1  "Steering IF Ang"
  Bus Creator1/1 -> Steer.IF/1
  Steering/2 -> Demux/1
  Bus Creator2/1 -> Terminator/1  "Steer IF (in)"
  VhclCtrl.Steering/1 -> Steering/2
  Steering/1 -> Sync_Out/1
  Sync_In/1 -> Steering/1

== system SD2231_Lab1_2022/CarMaker/IPG Vehicle/CarAndTrailer/Trailer ==
  Sync_In : Inport
  Trailer.Load : Inport  Port=2
  Car.Hitch : Inport  Port=3
  Car.Fr1 : Inport  Port=4
  Car.Trq_T2W : Inport  Port=5
  WheelCarrier.Misc : Inport  Port=6
  CreateBus Car.Hitch.FrcTrq : Subsystem
  CreateBus Vhcl.Motion : Subsystem
  CreateBus Vhcl.PoI : Subsystem
  CreateBus Vhcl.Steering : Subsystem
  CreateBus Vhcl.Wheel.FL : Subsystem
  CreateBus Vhcl.Wheel.FR : Subsystem
  CreateBus Vhcl.Wheel.RL : Subsystem
  CreateBus Vhcl.Wheel.RR : Subsystem
  Trailer : S-Function  FunctionName=CM_Sfun  Parameters='Trailer'  SFunctionDeploymentMode=off  EnableBusSupport=off
  Sync_Out : Outport
  Vhcl.Steering : Outport  Port=2
  Vhcl.Motion : Outport  Port=3
  Vhcl.PoI : Outport  Port=4
  Vhcl.Wheel.FL : Outport  Port=5
  Vhcl.Wheel.FR : Outport  Port=6
  Vhcl.Wheel.RL : Outport  Port=7
  Vhcl.Wheel.RR : Outport  Port=8
  Car.Hitch.FrcTrq : Outport  Port=9
  wires:
  Trailer/2 -> CreateBus Vhcl.Steering/1(In1)
  CreateBus Vhcl.Steering/1(Out1) -> Vhcl.Steering/1  "Vhcl.Steering"
  Trailer/3 -> CreateBus Vhcl.Motion/1(In1)
  Trailer/4 -> CreateBus Vhcl.PoI/1(In1)
  Trailer/5 -> CreateBus Vhcl.Wheel.FL/1(In1)
  Trailer/6 -> CreateBus Vhcl.Wheel.FR/1(In1)
  Trailer/7 -> CreateBus Vhcl.Wheel.RL/1(In1)
  Trailer/9 -> CreateBus Car.Hitch.FrcTrq/1(In1)
  Trailer/8 -> CreateBus Vhcl.Wheel.RR/1(In1)
  CreateBus Vhcl.Wheel.RR/1(Out1) -> Vhcl.Wheel.RR/1  "Vhcl.Wheel.RR"
  CreateBus Vhcl.Wheel.RL/1(Out1) -> Vhcl.Wheel.RL/1  "Vhcl.Wheel.RL"
  CreateBus Vhcl.Wheel.FR/1(Out1) -> Vhcl.Wheel.FR/1  "Vhcl.Wheel.FR"
  CreateBus Vhcl.Wheel.FL/1(Out1) -> Vhcl.Wheel.FL/1  "Vhcl.Wheel.FL"
  CreateBus Vhcl.PoI/1(Out1) -> Vhcl.PoI/1  "Vhcl.PoI"
  CreateBus Vhcl.Motion/1(Out1) -> Vhcl.Motion/1  "Vhcl.Motion"
  Car.Trq_T2W/1 -> Trailer/5
  WheelCarrier.Misc/1 -> Trailer/6
  CreateBus Car.Hitch.FrcTrq/1(Out1) -> Car.Hitch.FrcTrq/1  "Car.Hitch.FrcTrq"
  Car.Fr1/1 -> Trailer/4
  Car.Hitch/1 -> Trailer/3
  Trailer.Load/1 -> Trailer/2
  Trailer/1 -> Sync_Out/1
  Sync_In/1 -> Trailer/1

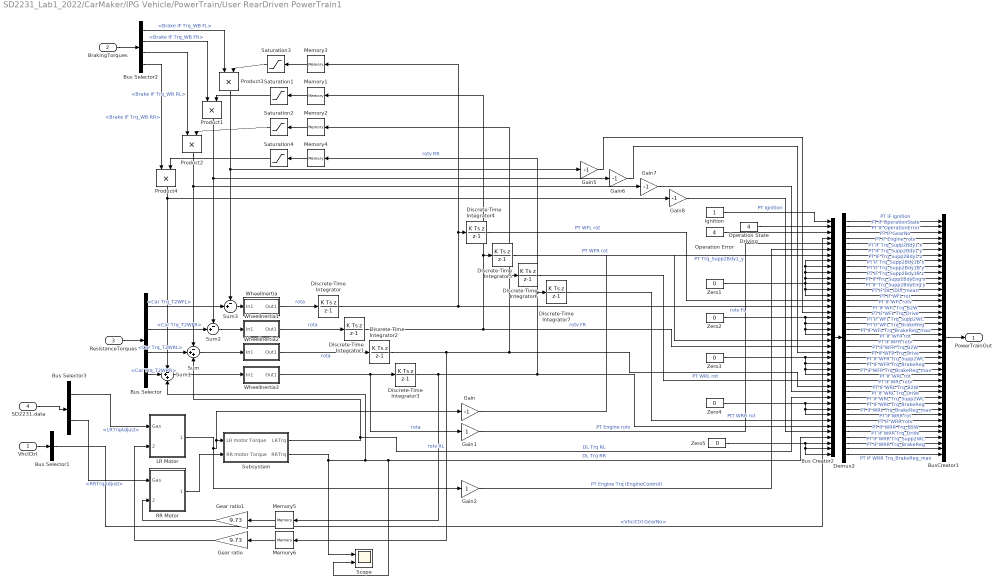
== system SD2231_Lab1_2022/CarMaker/IPG Vehicle/PowerTrain/User RearDriven PowerTrain1 ==
  VhclCtrl : Inport
  BrakingTorques : Inport  Port=2
  ResistanceTorques : Inport  Port=3
  SD2231.data : Inport  Port=4
  Bus Creator2 : BusCreator  Inputs=42
  Bus Selector : BusSelector  OutputSignals=Car Trq_T2WFL,Car Trq_T2WFR,Car Trq_T2WRL,Car Trq_T2WRR
  Bus Selector1 : BusSelector  OutputSignals=VhclCtrl GearNo
  Bus Selector2 : BusSelector  OutputSignals=Brake IF Trq_WB FL,Brake IF Trq_WB FR,Brake IF Trq_WB RL,Brake IF Trq_WB RR
  Bus Selector3 : BusSelector  OutputSignals=LRTrqAdjust,RRTrqAdjust
  BusCreator1 : BusCreator  Inputs=42
  Demux2 : Demux  Outputs=42
      settings: DisplayOption=none
  Discrete-Time Integrator{,1..7} (8 alike) : DiscreteIntegrator  IntegratorMethod=Integration: Backward Euler  SampleTime=0.001  ICPrevOutput=DiscIntNeverNeededParam  ICPrevScaledInput=DiscIntNeverNeededParam
  Gain{,5..8} (5 alike) : Gain  Gain=-1
      Gain settings: AttributesFormatString=%<Gain>
  Gain1 : Gain
      settings: AttributesFormatString=%<Gain>
  Gain2 : Gain
      settings: AttributesFormatString=%<Gain>
  Gear ratio : Gain  Gain=9.73
  Gear ratio1 : Gain  Gain=9.73
  Ignition : Constant
  LR Motor : Subsystem
  Memory{1..6} (6 alike) : Memory
  Operation Error : Constant  Value=4
  Operation State Driving : Constant  Value=4
  Product{1..4} (4 alike) : Product  RndMeth=Zero
  RR Motor : Subsystem
  Saturation{1..4} (4 alike) : Saturate  UpperLimit=1  LowerLimit=-1
  Scope : Scope  NumInputPorts=2
  Subsystem : Subsystem
  Sum : Sum  Inputs=-++
  Sum1 : Sum  Inputs=-++
  Sum2 : Sum  Inputs=-+|
  Sum3 : Sum  Inputs=-+|
  WheelInertia : Subsystem
  WheelInertia1 : Subsystem
  WheelInertia2 : Subsystem
  WheelInertia3 : Subsystem
  Zero{1..5} (5 alike) : Constant  Value=0
  PowerTrainOut : Outport  VectorParamsAs1DForOutWhenUnconnected=off
  wires:
  Saturation4/1 -> Product4/2
  Memory4/1 -> Saturation4/1
  Bus Selector2/4 -> Product4/1  "<Brake IF Trq_WB RR>"
  Product4/1 -> Sum1/1, Gain8/1
  Saturation2/1 -> Product2/2
  Memory2/1 -> Saturation2/1
  Bus Selector2/3 -> Product2/1  "<Brake IF Trq_WB RL>"
  Product2/1 -> Sum/1, Gain7/1
  Saturation1/1 -> Product1/2
  Memory1/1 -> Saturation1/1
  Bus Selector2/2 -> Product1/1  "<Brake IF Trq_WB FR>"
  Product1/1 -> Sum2/1, Gain6/1
  Memory3/1 -> Saturation3/1
  Saturation3/1 -> Product3/2
  Bus Selector2/1 -> Product3/1  "<Brake IF Trq_WB FL>"
  Product3/1 -> Sum3/1, Gain5/1
  BrakingTorques/1 -> Bus Selector2/1
  Sum3/1 -> WheelInertia/1(In1)
  Bus Selector/1 -> Sum3/2  "<Car Trq_T2WFL>"
  Sum2/1 -> WheelInertia1/1(In1)
  Bus Selector/4 -> Sum1/2  "<Car Trq_T2WRR>"
  Bus Selector/3 -> Sum/2  "<Car Trq_T2WRL>"
  Bus Selector1/1 -> Bus Creator2/4  "<VhclCtrl GearNo>"
  VhclCtrl/1 -> Bus Selector1/1
  LR Motor/1(Motor Trq) -> Gain2/1, Gain/1, Subsystem/1(LR motor Torque)
  Discrete-Time Integrator3/1 -> Memory5/1, Memory4/1, Discrete-Time Integrator7/1, Bus Creator2/37  "rotv RR"
  Discrete-Time Integrator/1 -> Memory3/1, Discrete-Time Integrator4/1, Bus Creator2/16  "rotv FL"
  Discrete-Time Integrator1/1 -> Memory1/1, Discrete-Time Integrator5/1, Bus Creator2/23  "rotv FR"
  Discrete-Time Integrator2/1 -> Memory6/1, Memory2/1, Discrete-Time Integrator6/1, Bus Creator2/30  "rotv RL"
  Sum1/1 -> WheelInertia3/1(In1)
  WheelInertia3/1(Out1) -> Gain1/1, Discrete-Time Integrator3/1  "rota"
  Sum/1 -> WheelInertia2/1(In1)
  WheelInertia2/1(Out1) -> Discrete-Time Integrator2/1  "rota"
  Bus Selector/2 -> Sum2/2  "<Car Trq_T2WFR>"
  WheelInertia1/1(Out1) -> Discrete-Time Integrator1/1  "rota"
  ResistanceTorques/1 -> Bus Selector/1
  WheelInertia/1(Out1) -> Discrete-Time Integrator/1  "rota"
  Gain/1 -> Bus Creator2/7  "PT Trq_Supp2Bdy1_y"
  Gain1/1 -> Bus Creator2/5  "PT Engine rotv"
  Gain2/1 -> Bus Creator2/6  "PT Engine Trq (EngineControl)"
  Discrete-Time Integrator7/1 -> Bus Creator2/36  "PtT WRR rot"
  Discrete-Time Integrator6/1 -> Bus Creator2/29  "PT WRL rot"
  Discrete-Time Integrator5/1 -> Bus Creator2/22  "PT WFR rot"
  Discrete-Time Integrator4/1 -> Bus Creator2/15  "PT WFL rot"
  Ignition/1 -> Bus Creator2/1  "PT Ignition"
  Bus Creator2/1 -> Demux2/1
  Operation State Driving/1 -> Bus Creator2/2
  Operation Error/1 -> Bus Creator2/3
  Zero1/1 -> Bus Creator2/12, Bus Creator2/14, Bus Creator2/13, Bus Creator2/11, Bus Creator2/10, Bus Creator2/9, Bus Creator2/8
  Zero2/1 -> Bus Creator2/19, Bus Creator2/20, Bus Creator2/21, Bus Creator2/18
  Zero3/1 -> Bus Creator2/26, Bus Creator2/27, Bus Creator2/28, Bus Creator2/25
  Zero4/1 -> Bus Creator2/33, Bus Creator2/34, Bus Creator2/35
  Zero5/1 -> Bus Creator2/40, Bus Creator2/41, Bus Creator2/42
  Subsystem/1("LRTrq ") -> Bus Creator2/32, Sum/3  "DL Trq RL"
  Gain6/1 -> Bus Creator2/24
  Gain5/1 -> Bus Creator2/17
  Gain7/1 -> Bus Creator2/31
  Gain8/1 -> Bus Creator2/38
  Demux2/42 -> BusCreator1/42  "PT IF WRR Trq_BrakeReg_max"
  Demux2/41 -> BusCreator1/41  "PT IF WRR Trq_BrakeReg"
  Demux2/40 -> BusCreator1/40  "PT IF WRR Trq_Supp2WC"
  Demux2/39 -> BusCreator1/39  "PT IF WRR Trq_Drive"
  Demux2/38 -> BusCreator1/38  "PT IF WRR Trq_B2W"
  Demux2/37 -> BusCreator1/37  "PT IF WRR rotv"
  Demux2/36 -> BusCreator1/36  "PT IF WRR rot"
  Demux2/35 -> BusCreator1/35  "PT IF WRL Trq_BrakeReg_max"
  Demux2/34 -> BusCreator1/34  "PT IF WRL Trq_BrakeReg"
  Demux2/33 -> BusCreator1/33  "PT IF WRL Trq_Supp2WC"
  Demux2/32 -> BusCreator1/32  "PT IF WRL Trq_Drive"
  Demux2/31 -> BusCreator1/31  "PT IF WRL Trq_B2W"
  Demux2/30 -> BusCreator1/30  "PT IF WRL rotv"
  Demux2/29 -> BusCreator1/29  "PT IF WRL rot"
  Demux2/28 -> BusCreator1/28  "PT IF WFR Trq_BrakeReg_max"
  Demux2/27 -> BusCreator1/27  "PT IF WFR Trq_BrakeReg"
  Demux2/26 -> BusCreator1/26  "PT IF WFR Trq_Supp2WC"
  Demux2/25 -> BusCreator1/25  "PT IF WFR Trq_Drive"
  Demux2/24 -> BusCreator1/24  "PT IF WFR Trq_B2W"
  Demux2/23 -> BusCreator1/23  "PT IF WFR rotv"
  Demux2/22 -> BusCreator1/22  "PT IF WFR rot"
  Demux2/21 -> BusCreator1/21  "PT IF WFL Trq_BrakeReg_max"
  Demux2/20 -> BusCreator1/20  "PT IF WFL Trq_BrakeReg"
  Demux2/19 -> BusCreator1/19  "PT IF WFL Trq_Supp2WC"
  Demux2/18 -> BusCreator1/18  "PT IF WFL Trq_Drive"
  Demux2/17 -> BusCreator1/17  "PT IF WFL Trq_B2W"
  Demux2/16 -> BusCreator1/16  "PT IF WFL rotv"
  Demux2/15 -> BusCreator1/15  "PT IF WFL rot"
  Demux2/14 -> BusCreator1/14  "PT IF DL_iDiff_mean"
  Demux2/13 -> BusCreator1/13  "PT IF Trq_Supp2BdyEng y"
  Demux2/12 -> BusCreator1/12  "PT IF Trq_Supp2BdyEng x"
  Demux2/11 -> BusCreator1/11  "PT IF Trq_Supp2Bdy1B z"
  Demux2/10 -> BusCreator1/10  "PT IF Trq_Supp2Bdy1B y"
  Demux2/9 -> BusCreator1/9  "PT IF Trq_Supp2Bdy1B x"
  Demux2/8 -> BusCreator1/8  "PT IF Trq_Supp2Bdy1 z"
  Demux2/7 -> BusCreator1/7  "PT IF Trq_Supp2Bdy1 y"
  Demux2/6 -> BusCreator1/6  "PT IF Trq_Supp2Bdy1 x"
  Demux2/5 -> BusCreator1/5  "PT IF Engine_rotv"
  Demux2/4 -> BusCreator1/4  "PT IF GearNo"
  Demux2/3 -> BusCreator1/3  "PT IF OperationError"
  Demux2/2 -> BusCreator1/2  "PT IF OperationState"
  Demux2/1 -> BusCreator1/1  "PT IF Ignition"
  BusCreator1/1 -> PowerTrainOut/1
  Memory5/1 -> Gear ratio1/1
  Subsystem/2(RRTrq) -> Scope/1, Scope/2, Bus Creator2/39, Sum1/3  "DL Trq RR"
  SD2231.data/1 -> Bus Selector3/1
  Bus Selector3/1 -> LR Motor/1(Gas)  "<LRTrqAdjust>"
  RR Motor/1(Motor Trq) -> Subsystem/2(RR motor Torque)
  Bus Selector3/2 -> RR Motor/1(Gas)  "<RRTrqAdjust>"
  Memory6/1 -> Gear ratio/1
  Gear ratio/1 -> LR Motor/2("Motor speed ")
  Gear ratio1/1 -> RR Motor/2("Motor speed ")

== system SD2231_Lab1_2022/CarMaker/Your ABS Controller/Activation Logic Br FL/Subsystem ==
  slip : Inport
  ref_slip : Inport  Port=2
  Brake Pedal : Inport  Port=3
  AdjBr FL : Scope
  PID1 : Subsystem
      settings: PortSchema="{\"entries\":[{\"content\":{\"sides\":[{\"content\":{\"connectorIds\":[\"In1\"]},\"type\":\"ConnectorPlacement.EquallySpacedRectSide\",\"uuid\":\"a0a678af-e4e1-4120-b7ef-0ef542f8e9cc\"},{\"content\":{\"connectorIds\":[\"Out1\"],\"side\":\"RIGHT\"},\"type\":\"ConnectorPlacement.EquallySpacedRectSide\",\"uuid\":\"903d0154-0882-4438-b528-a9d871d2aaef\"},{\"content\":{\"connectorIds\":[],\"side\":\"TOP\"},\"type\":\"ConnectorPlacement.EquallySpacedRectSide\",\"uuid\":\"cc0bbc94-fd35-44a3-99eb-327b952e9968\"},{\"content\":{\"connectorIds\":[\"In2\",\"In3\"],\"side\":\"BOTTOM\"},\"type\":\"ConnectorPlacement.EquallySpacedRectSide\",\"uuid\":\"05665a86-e33a-4510-a8ad-b2cae5a94577\"},{\"content\":{\"connectorIds\":[],\"side\":\"HIDDEN\"},\"type\":\"ConnectorPlacement.EquallySpacedRectSide\",\"uuid\":\"9e1bf206-7ec4-44f3-a0bc-dd9892acac44\"}]},\"type\":\"ConnectorPlacement.EquallySpacedConnector\",\"uuid\":\"274c0393-67a6-46bd-bc80-41d54c35eeb8\"}],\"packageUris\":[\"http://schema.mathworks.com/mf0/Connector/R2020b\"],\"version\":\"1.0\"}"
  Subtract : Sum  Inputs=+-
  err Br FL : Scope
  AdjThr : Outport
  wires:
  PID1/1(AdjBrk) -> AdjBr FL/1, AdjThr/1  "AdjTh"
  slip/1 -> PID1/3(slip), Subtract/2
  ref_slip/1 -> Subtract/1
  Subtract/1 -> PID1/1(err)  "err_slip"
  Brake Pedal/1 -> PID1/2(Brake Pedal)

== system SD2231_Lab1_2022/CarMaker/Your ABS Controller/Activation Logic Br FR/Subsystem ==
  slip : Inport
  ref_slip : Inport  Port=2
  Brake Pedal : Inport  Port=3
  MATLAB Function : MATLAB Function  TreatAsAtomicUnit=on
  PID : Subsystem
      settings: PortSchema="{\"entries\":[{\"content\":{\"sides\":[{\"content\":{\"connectorIds\":[\"In1\"]},\"type\":\"ConnectorPlacement.EquallySpacedRectSide\",\"uuid\":\"4085cc8c-76f8-4571-b5c6-610b0576e246\"},{\"content\":{\"connectorIds\":[\"Out1\"],\"side\":\"RIGHT\"},\"type\":\"ConnectorPlacement.EquallySpacedRectSide\",\"uuid\":\"af62d16b-21fe-47cd-97ad-a8be9811ce56\"},{\"content\":{\"connectorIds\":[\"In2\"],\"side\":\"TOP\"},\"type\":\"ConnectorPlacement.EquallySpacedRectSide\",\"uuid\":\"cce2fb25-5446-4832-92f9-d88aea361fa1\"},{\"content\":{\"connectorIds\":[],\"side\":\"HIDDEN\"},\"type\":\"ConnectorPlacement.EquallySpacedRectSide\",\"uuid\":\"539ad2f7-bc65-45dc-9658-2db591c9cd5f\"}]},\"type\":\"ConnectorPlacement.EquallySpacedConnector\",\"uuid\":\"aba1dd86-6cf6-453e-9027-1859e3ca8db9\"}],\"packageUris\":[\"http://schema.mathworks.com/mf0/Connector/R2020b\"],\"version\":\"1.0\"}"
  Subtract : Sum  Inputs=+-
  AdjThr : Outport
  wires:
  ref_slip/1 -> Subtract/1
  slip/1 -> Subtract/2
  Subtract/1 -> PID/1(err)  "err_slip"
  PID/1(Out1) -> AdjThr/1  "AdjTh"
  Brake Pedal/1 -> MATLAB Function/1(Brk)
  MATLAB Function/1(res) -> PID/2(res)

== system SD2231_Lab1_2022/CarMaker/Your ABS Controller/Activation Logic Br FR/Subsystem1 ==
  slip : Inport
  ref_slip : Inport  Port=2
  Brake Pedal : Inport  Port=3
  AdjBr FL : Scope
  PID1 : Subsystem
      settings: PortSchema="{\"entries\":[{\"content\":{\"sides\":[{\"content\":{\"connectorIds\":[\"In1\"]},\"type\":\"ConnectorPlacement.EquallySpacedRectSide\",\"uuid\":\"a0a678af-e4e1-4120-b7ef-0ef542f8e9cc\"},{\"content\":{\"connectorIds\":[\"Out1\"],\"side\":\"RIGHT\"},\"type\":\"ConnectorPlacement.EquallySpacedRectSide\",\"uuid\":\"903d0154-0882-4438-b528-a9d871d2aaef\"},{\"content\":{\"connectorIds\":[],\"side\":\"TOP\"},\"type\":\"ConnectorPlacement.EquallySpacedRectSide\",\"uuid\":\"cc0bbc94-fd35-44a3-99eb-327b952e9968\"},{\"content\":{\"connectorIds\":[\"In2\",\"In3\"],\"side\":\"BOTTOM\"},\"type\":\"ConnectorPlacement.EquallySpacedRectSide\",\"uuid\":\"05665a86-e33a-4510-a8ad-b2cae5a94577\"},{\"content\":{\"connectorIds\":[],\"side\":\"HIDDEN\"},\"type\":\"ConnectorPlacement.EquallySpacedRectSide\",\"uuid\":\"9e1bf206-7ec4-44f3-a0bc-dd9892acac44\"}]},\"type\":\"ConnectorPlacement.EquallySpacedConnector\",\"uuid\":\"274c0393-67a6-46bd-bc80-41d54c35eeb8\"}],\"packageUris\":[\"http://schema.mathworks.com/mf0/Connector/R2020b\"],\"version\":\"1.0\"}"
  Subtract : Sum  Inputs=+-
  err Br FL : Scope
  AdjThr : Outport
  wires:
  Brake Pedal/1 -> PID1/2(Brake Pedal)
  PID1/1(AdjBrk) -> AdjBr FL/1, AdjThr/1  "AdjTh"
  Subtract/1 -> PID1/1(err), err Br FL/1  "err_slip"
  slip/1 -> PID1/3(slip), Subtract/2
  ref_slip/1 -> Subtract/1

== system SD2231_Lab1_2022/CarMaker/Your ABS Controller/Activation Logic Br RL/Subsystem ==
  slip : Inport
  ref_slip : Inport  Port=2
  Brake Pedal : Inport  Port=3
  AdjBr RL : Scope
  PID1 : Subsystem
      settings: PortSchema="{\"entries\":[{\"content\":{\"sides\":[{\"content\":{\"connectorIds\":[\"In1\"]},\"type\":\"ConnectorPlacement.EquallySpacedRectSide\",\"uuid\":\"a0a678af-e4e1-4120-b7ef-0ef542f8e9cc\"},{\"content\":{\"connectorIds\":[\"Out1\"],\"side\":\"RIGHT\"},\"type\":\"ConnectorPlacement.EquallySpacedRectSide\",\"uuid\":\"903d0154-0882-4438-b528-a9d871d2aaef\"},{\"content\":{\"connectorIds\":[],\"side\":\"TOP\"},\"type\":\"ConnectorPlacement.EquallySpacedRectSide\",\"uuid\":\"cc0bbc94-fd35-44a3-99eb-327b952e9968\"},{\"content\":{\"connectorIds\":[\"In2\",\"In3\"],\"side\":\"BOTTOM\"},\"type\":\"ConnectorPlacement.EquallySpacedRectSide\",\"uuid\":\"05665a86-e33a-4510-a8ad-b2cae5a94577\"},{\"content\":{\"connectorIds\":[],\"side\":\"HIDDEN\"},\"type\":\"ConnectorPlacement.EquallySpacedRectSide\",\"uuid\":\"9e1bf206-7ec4-44f3-a0bc-dd9892acac44\"}]},\"type\":\"ConnectorPlacement.EquallySpacedConnector\",\"uuid\":\"274c0393-67a6-46bd-bc80-41d54c35eeb8\"}],\"packageUris\":[\"http://schema.mathworks.com/mf0/Connector/R2020b\"],\"version\":\"1.0\"}"
  Subtract : Sum  Inputs=+-
  AdjThr : Outport
  wires:
  PID1/1(AdjBrk) -> AdjBr RL/1, AdjThr/1  "AdjTh"
  slip/1 -> PID1/2(slip), Subtract/2
  ref_slip/1 -> Subtract/1
  Subtract/1 -> PID1/1(err)  "err_slip"
  Brake Pedal/1 -> PID1/3(Brake Pedal)

== system SD2231_Lab1_2022/CarMaker/Your ABS Controller/Activation Logic Br RL old/Subsystem ==
  slip : Inport
  ref_slip : Inport  Port=2
  Brake Pedal : Inport  Port=3
  MATLAB Function : MATLAB Function  TreatAsAtomicUnit=on
  PID : Subsystem
      settings: PortSchema="{\"entries\":[{\"content\":{\"sides\":[{\"content\":{\"connectorIds\":[\"In1\"]},\"type\":\"ConnectorPlacement.EquallySpacedRectSide\",\"uuid\":\"4085cc8c-76f8-4571-b5c6-610b0576e246\"},{\"content\":{\"connectorIds\":[\"Out1\"],\"side\":\"RIGHT\"},\"type\":\"ConnectorPlacement.EquallySpacedRectSide\",\"uuid\":\"af62d16b-21fe-47cd-97ad-a8be9811ce56\"},{\"content\":{\"connectorIds\":[\"In2\"],\"side\":\"TOP\"},\"type\":\"ConnectorPlacement.EquallySpacedRectSide\",\"uuid\":\"cce2fb25-5446-4832-92f9-d88aea361fa1\"},{\"content\":{\"connectorIds\":[],\"side\":\"HIDDEN\"},\"type\":\"ConnectorPlacement.EquallySpacedRectSide\",\"uuid\":\"539ad2f7-bc65-45dc-9658-2db591c9cd5f\"}]},\"type\":\"ConnectorPlacement.EquallySpacedConnector\",\"uuid\":\"aba1dd86-6cf6-453e-9027-1859e3ca8db9\"}],\"packageUris\":[\"http://schema.mathworks.com/mf0/Connector/R2020b\"],\"version\":\"1.0\"}"
  Subtract : Sum  Inputs=+-
  err Br RL : Scope
  AdjThr : Outport
  wires:
  ref_slip/1 -> Subtract/1
  slip/1 -> Subtract/2
  Subtract/1 -> err Br RL/1, PID/1(err)  "err_slip"
  PID/1(Out1) -> AdjThr/1  "AdjTh"
  Brake Pedal/1 -> MATLAB Function/1(Brk)
  MATLAB Function/1(res) -> PID/2(res)

== system SD2231_Lab1_2022/CarMaker/Your ABS Controller/Activation Logic Br RL old 2/Controller ==
  slip : Inport
  ref_slip : Inport  Port=2
  Brake Pedal : Inport  Port=3
  AdjBrk RL : Scope
  PID : Subsystem
      settings: PortSchema="{\"entries\":[{\"content\":{\"sides\":[{\"content\":{\"connectorIds\":[\"In1\"]},\"type\":\"ConnectorPlacement.EquallySpacedRectSide\",\"uuid\":\"a0a678af-e4e1-4120-b7ef-0ef542f8e9cc\"},{\"content\":{\"connectorIds\":[\"Out1\"],\"side\":\"RIGHT\"},\"type\":\"ConnectorPlacement.EquallySpacedRectSide\",\"uuid\":\"903d0154-0882-4438-b528-a9d871d2aaef\"},{\"content\":{\"connectorIds\":[],\"side\":\"TOP\"},\"type\":\"ConnectorPlacement.EquallySpacedRectSide\",\"uuid\":\"cc0bbc94-fd35-44a3-99eb-327b952e9968\"},{\"content\":{\"connectorIds\":[\"In2\"],\"side\":\"BOTTOM\"},\"type\":\"ConnectorPlacement.EquallySpacedRectSide\",\"uuid\":\"05665a86-e33a-4510-a8ad-b2cae5a94577\"},{\"content\":{\"connectorIds\":[],\"side\":\"HIDDEN\"},\"type\":\"ConnectorPlacement.EquallySpacedRectSide\",\"uuid\":\"9e1bf206-7ec4-44f3-a0bc-dd9892acac44\"}]},\"type\":\"ConnectorPlacement.EquallySpacedConnector\",\"uuid\":\"274c0393-67a6-46bd-bc80-41d54c35eeb8\"}],\"packageUris\":[\"http://schema.mathworks.com/mf0/Connector/R2020b\"],\"version\":\"1.0\"}"
  Subtract : Sum  Inputs=+-
  Transfer Fcn : TransferFcn  Commented=through  Denominator=[1 0.1]
  err Br RL : Scope
  AdjThr : Outport
  wires:
  ref_slip/1 -> Subtract/1
  slip/1 -> Subtract/2
  PID/1(AdjBrk) -> AdjThr/1, AdjBrk RL/1  "AdjTh"
  Transfer Fcn/1 -> PID/1(err), err Br RL/1
  Brake Pedal/1 -> PID/2(Brake Pedal)
  Subtract/1 -> Transfer Fcn/1  "err_slip"
